simulink model "robtik1"  (Simulink 9.0)
settings: Solver=ode45  StartTime=0.0  StopTime=999999  MaxStep=10  MinStep=0.0001  RelTol=1e-3  AbsTol=1e-3  EnableMultiTasking=on
undefined symbols (not defined in the file or in its folder): a4, d1
settings Model: Creator=Anders  LastModifiedBy=esmu
settings DataIOCC: LimitDataPoints=on  SignalLoggingSaveFormat=ModelDataLogs  SaveOutput=off  SaveTime=off  SignalLoggingName=sigsOut
settings OptimizationCC: ExpressionDepthLimit=2147483647  InitFltsAndDblsToZero=on
settings DebuggingCC: SaveWithParameterizedLinksMsg=none  SignalResolutionControl=TryResolveAllWithWarning  MultiTaskDSMMsg=warning  MultiTaskCondExecSysMsg=none  FcnCallInpInsideContextMsg=warning  StateNameClashWarn=warning  StrictBusMsg=None
settings HardwareCC: TargetUnknown=on
settings GRTTargetCC: TargetFcnLib=ansi_tfl_tmw.mat  GeneratePreprocessorConditionals=Disable all  CombineOutputUpdateFcns=off  GRTInterface=on

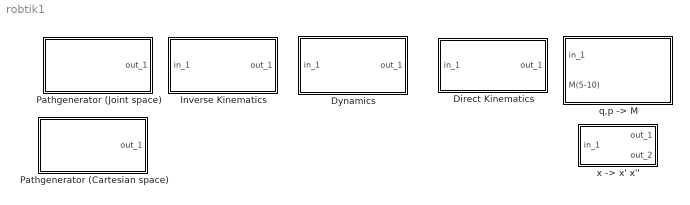
== system robtik1 ==
  Direct Kinematics : Subsystem
      mask Display: disp('Alto-Robot')
  Dynamics : Subsystem
      mask Display: disp('Alto-Robot\n tau -> q,q''')
  Inverse Kinematics : Subsystem
      mask Display: disp('Alto-Robot')
  "Pathgenerator (Cartesian space) " : Subsystem
      mask Display: disp('Alto-Robot\nPath -> p')
  Pathgenerator (Joint space) : Subsystem
      mask Display: disp('Alto-Robot\n path -> q')
  "q,p -> M" : Subsystem
      mask Display: disp('Save to vis4link')
  "x -> x' x''" : Subsystem
      mask Display: disp('Vector diff.')

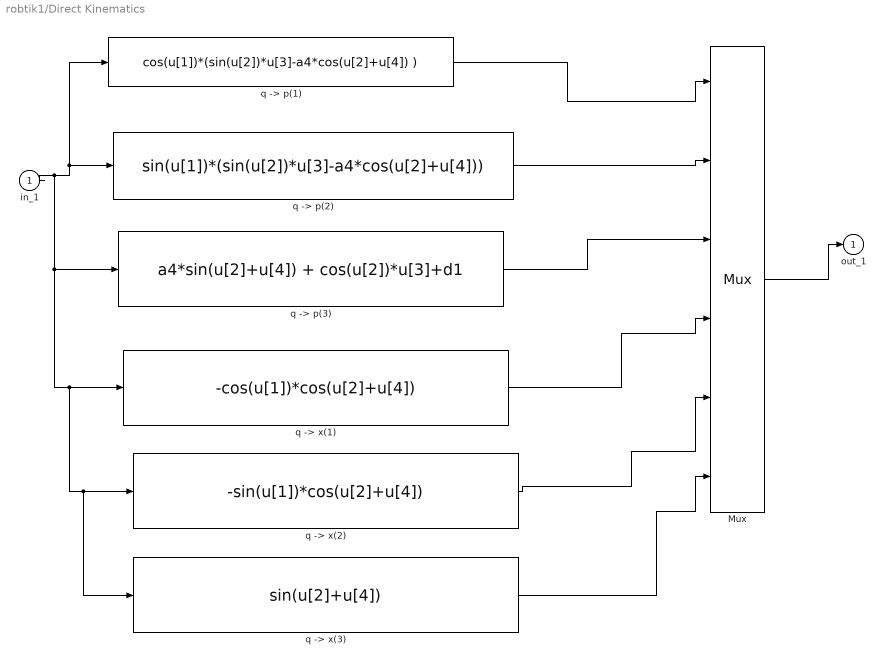
== system robtik1/Direct Kinematics ==
  in_1 : Inport
  Mux : Mux  Inputs=6
  "q -> p(1)" : Fcn  Expr=cos(u[1])*(sin(u[2])*u[3]-a4*cos(u[2]+u[4]) )
  "q -> p(2)" : Fcn  Expr=sin(u[1])*(sin(u[2])*u[3]-a4*cos(u[2]+u[4]))
  "q -> p(3)" : Fcn  Expr=a4*sin(u[2]+u[4]) + cos(u[2])*u[3]+d1
  "q -> x(1)" : Fcn  Expr=-cos(u[1])*cos(u[2]+u[4])
  "q -> x(2)" : Fcn  Expr=-sin(u[1])*cos(u[2]+u[4])
  "q -> x(3)" : Fcn  Expr=sin(u[2]+u[4])
  out_1 : Outport  InitialOutput=0
  wires:
  Mux/1 -> out_1/1
  in_1/1 -> "q -> x(3)"/1, "q -> x(2)"/1, "q -> x(1)"/1, "q -> p(3)"/1, "q -> p(2)"/1, "q -> p(1)"/1
  "q -> x(3)"/1 -> Mux/6
  "q -> x(2)"/1 -> Mux/5
  "q -> x(1)"/1 -> Mux/4
  "q -> p(1)"/1 -> Mux/1
  "q -> p(2)"/1 -> Mux/2
  "q -> p(3)"/1 -> Mux/3

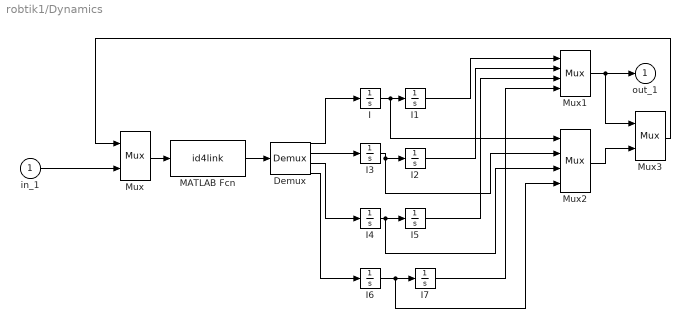
== system robtik1/Dynamics ==
  in_1 : Inport
  Demux : Demux
  I{,1..7} (8 alike) : Integrator
  MATLAB Fcn : MATLABFcn  MATLABFcn=id4link  OutputDimensions=4
  Mux : Mux  Inputs=[8 4]
  Mux1 : Mux
  Mux2 : Mux
  Mux3 : Mux  Inputs=[4 4]
  out_1 : Outport
  wires:
  in_1/1 -> Mux/2
  Mux2/1 -> Mux3/2
  I7/1 -> Mux1/4
  Demux/4 -> I6/1
  I6/1 -> Mux2/4, I7/1
  Mux/1 -> MATLAB Fcn/1
  MATLAB Fcn/1 -> Demux/1
  Demux/1 -> I/1
  I/1 -> I1/1, Mux2/1
  I3/1 -> I2/1, Mux2/2
  Demux/2 -> I3/1
  I4/1 -> I5/1, Mux2/3
  Demux/3 -> I4/1
  I2/1 -> Mux1/2
  I5/1 -> Mux1/3
  I1/1 -> Mux1/1
  Mux3/1 -> Mux/1
  Mux1/1 -> Mux3/1, out_1/1

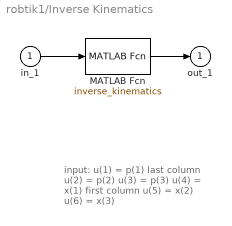
== system robtik1/Inverse Kinematics ==
  note: input:
      | u(1) = p(1) last column
      | u(2) = p(2)
      | u(3) = p(3)
      | u(4) = x(1) first column
      | u(5) = x(2)
      | u(6) = x(3)
  in_1 : Inport
  MATLAB Fcn : MATLABFcn  MATLABFcn=inverse_kinematics  OutputDimensions=4
  out_1 : Outport
  wires:
  MATLAB Fcn/1 -> out_1/1
  in_1/1 -> MATLAB Fcn/1

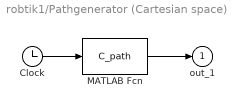
== system robtik1/Pathgenerator (Cartesian space)  ==
  Clock : Clock
  MATLAB Fcn : MATLABFcn  MATLABFcn=C_path  OutputDimensions=6
  out_1 : Outport
  wires:
  Clock/1 -> MATLAB Fcn/1
  MATLAB Fcn/1 -> out_1/1

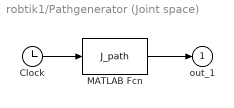
== system robtik1/Pathgenerator (Joint space) ==
  Clock : Clock
  MATLAB Fcn : MATLABFcn  MATLABFcn=J_path  OutputDimensions=4
  out_1 : Outport
  wires:
  MATLAB Fcn/1 -> out_1/1
  Clock/1 -> MATLAB Fcn/1

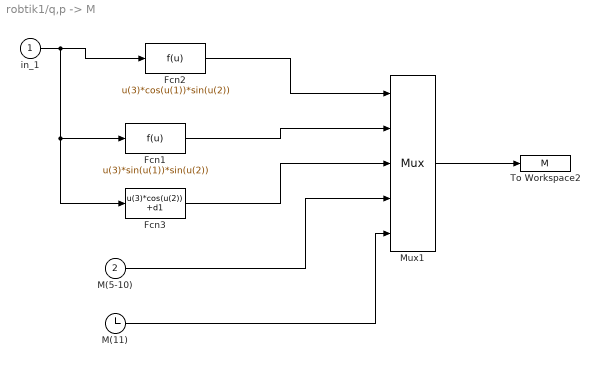
== system robtik1/q,p -> M ==
  in_1 : Inport
  M(5-10) : Inport  Port=2
  Fcn1 : Fcn  Expr=u(3)*sin(u(1))*sin(u(2))
  Fcn2 : Fcn  Expr=u(3)*cos(u(1))*sin(u(2))
  Fcn3 : Fcn  Expr=u(3)*cos(u(2)) +d1
  M(11) : Clock
  Mux1 : Mux  Inputs=[1 1 1 6 1]
  To Workspace2 : ToWorkspace  VariableName=M
      settings: MaxDataPoints=100000
  wires:
  M(11)/1 -> Mux1/5
  M(5-10)/1 -> Mux1/4
  Fcn3/1 -> Mux1/3
  Fcn1/1 -> Mux1/2
  Fcn2/1 -> Mux1/1
  in_1/1 -> Fcn3/1, Fcn1/1, Fcn2/1
  Mux1/1 -> To Workspace2/1

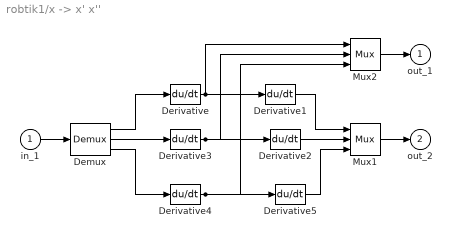
== system robtik1/x -> x' x'' ==
  in_1 : Inport
  Demux : Demux  Outputs=3
  Derivative{,1..5} (6 alike) : Derivative
  Mux1 : Mux  Inputs=3
  Mux2 : Mux  Inputs=3
  out_1 : Outport
  out_2 : Outport  Port=2
  wires:
  Mux1/1 -> out_2/1
  in_1/1 -> Demux/1
  Mux2/1 -> out_1/1
  Derivative/1 -> Derivative1/1, Mux2/1
  Derivative1/1 -> Mux1/1
  Derivative3/1 -> Derivative2/1, Mux2/2
  Derivative4/1 -> Derivative5/1, Mux2/3
  Derivative2/1 -> Mux1/2
  Derivative5/1 -> Mux1/3
  Demux/1 -> Derivative/1
  Demux/2 -> Derivative3/1
  Demux/3 -> Derivative4/1
